simulink model "Math2"  (R2017b)
settings: Solver=FixedStepDiscrete  StartTime=0.0  StopTime=10.0  FixedStep=0.200000  RelTol=1e-3  EnableMultiTasking=on
settings Model: Creator=ktrinh  LastModifiedBy=hbourbou
settings OptimizationCC: DefaultParameterBehavior=Inlined  LifeSpan=1
settings DebuggingCC: SFUnexpectedBacktrackingDiag=warning  SFNoUnconditionalDefaultTransitionDiag=warning  SFExecutionAtInitializationDiag=none
settings HardwareCC: ProdBitPerSizeT=32  ProdBitPerPtrDiffT=32  ProdWordSize=32  ProdHWDeviceType=Specified
settings SFSimCC: MATLABDynamicMemAlloc=off
settings RTWCC: SystemTargetFile=ert.tlc  TemplateMakefile=ert_default_tmf
settings CodeAppCC: IgnoreCustomStorageClasses=off  StateflowObjectComments=on
settings ERTTargetCC: MultiwordLength=2048  GenerateSampleERTMain=on  InlinedParameterPlacement=NonHierarchical  ERTCustomFileTemplate=example_file_process.tlc  ConvertIfToSwitch=off  SuppressUnreachableDefaultCases=off
settings ConfigComp: CovMetricSettings=dw  CovHtmlReporting=on  CovSaveCumulativeToWorkspaceVar=on  CovSaveSingleToWorkspaceVar=on  CovExternalEMLEnable=off

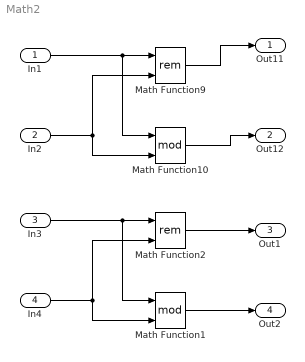
== system Math2 ==
  In1 : Inport
  In2 : Inport  Port=2
  In3 : Inport  Port=3  OutDataTypeStr=int32
  In4 : Inport  Port=4  OutDataTypeStr=int32
  Math Function1 : Math  Operator=mod  SaturateOnIntegerOverflow=on
  Math Function10 : Math  Operator=mod  SaturateOnIntegerOverflow=on
  Math Function2 : Math  Operator=rem  SaturateOnIntegerOverflow=on
  Math Function9 : Math  Operator=rem  SaturateOnIntegerOverflow=on
  Out11 : Outport
  Out12 : Outport  Port=2
  Out1 : Outport  Port=3
  Out2 : Outport  Port=4
  wires:
  In1/1 -> Math Function10/1, Math Function9/1
  Math Function9/1 -> Out11/1
  Math Function10/1 -> Out12/1
  In2/1 -> Math Function9/2, Math Function10/2
  In3/1 -> Math Function1/1, Math Function2/1
  Math Function2/1 -> Out1/1
  Math Function1/1 -> Out2/1
  In4/1 -> Math Function2/2, Math Function1/2
